simulink model "LinearMap"  (R2023b)
settings: configuration reference "Run_on_Hardware_Configuration" (kept outside this file)
settings Model: DataDictionary=SharedData.sldd  FPTRunName=Active  ExtModeTrigDuration=2  Creator=Tyler  LastModifiedBy=Tyler
settings ConfigSetRef: SourceName=Run_on_Hardware_Configuration

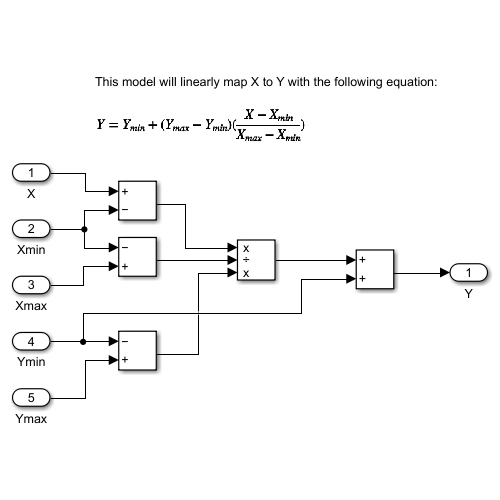
[thumbnail: Simulink's stored preview of the top-level diagram]
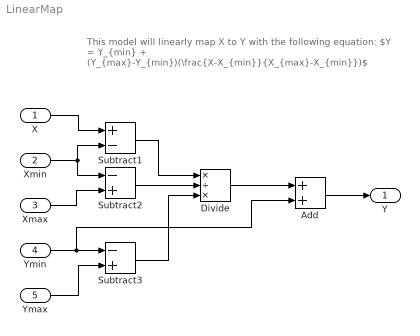
== system LinearMap ==
  note: This model will linearly map X to Y with the following equation:
      |
      | $Y = Y_{min} + (Y_{max}-Y_{min})(\frac{X-X_{min}}{X_{max}-X_{min}})$
  X : Inport
  Xmin : Inport  Port=2
  Xmax : Inport  Port=3
  Ymin : Inport  Port=4
  Ymax : Inport  Port=5
  Add : Sum
  Divide : Product  Inputs=*/*
  Subtract1 : Sum  Inputs=+-
  Subtract2 : Sum  Inputs=-+
  Subtract3 : Sum  Inputs=-+
  Y : Outport
  wires:
  Xmin/1 -> Subtract2/1, Subtract1/2
  Ymax/1 -> Subtract3/2
  Xmax/1 -> Subtract2/2
  Subtract3/1 -> Divide/3
  X/1 -> Subtract1/1
  Divide/1 -> Add/1
  Subtract1/1 -> Divide/1
  Subtract2/1 -> Divide/2
  Ymin/1 -> Add/2, Subtract3/1
  Add/1 -> Y/1
